simulink model "fftuntitled"  (R2017a)
settings: Solver=VariableStepAuto  StartTime=0.0  StopTime=30  RelTol=1e-3
settings Model: Creator=eduardo  LastModifiedBy=eduardo

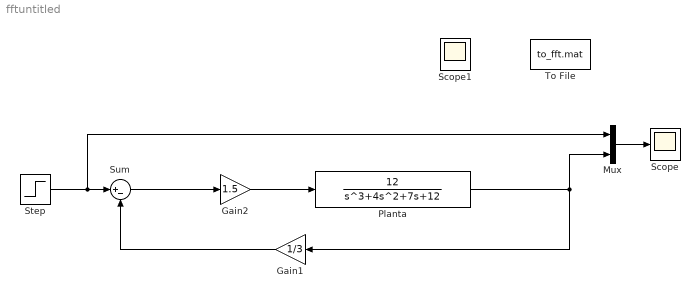
== system fftuntitled ==
  Gain1 : Gain  Gain=1/3
  Gain2 : Gain  Gain=1.5
  Mux : Mux  Inputs=2
  Planta : TransferFcn  Numerator=[12]  Denominator=[1 4 7 12]
  Scope : Scope
  Scope1 : Scope
  Step : Step  Time=2  SampleTime=0
  Sum : Sum  Inputs=|+-
  To File : ToFile  Filename=to_fft.mat  SaveFormat=Timeseries
  wires:
  Planta/1 -> Mux/2, Gain1/1
  Sum/1 -> Gain2/1
  Mux/1 -> Scope/1
  Step/1 -> Mux/1, Sum/1
  Gain1/1 -> Sum/2
  Gain2/1 -> Planta/1
